simulink model "PlantWateringProject"  (R2024a)
settings: Solver=VariableStepAuto  StartTime=0.0  StopTime=120.0  RelTol=1e-3
settings Model: Creator=charlieperkins  LastModifiedBy=charlieperkins

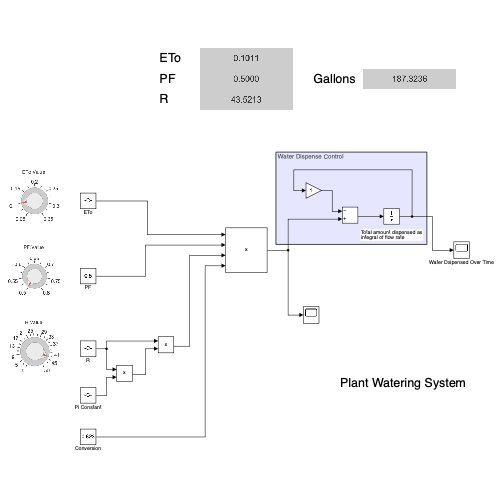
[thumbnail: Simulink's stored preview of the top-level diagram]
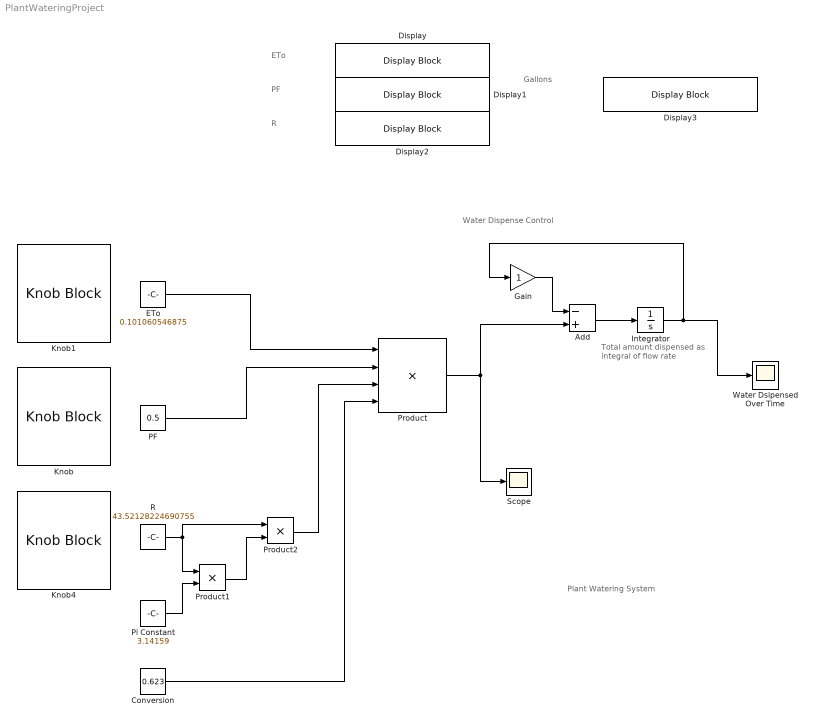
== system PlantWateringProject ==
  note: Water Dispense Control
  note: Total amount dispensed as
      | integral of flow rate
  note: ETo
  note: PF
  note: R
  note: Gallons
  note: Plant Watering System
  Add : Sum  Inputs=-+
  Conversion : Constant  Value=0.623
  Display{,1..3} (4 alike) : DisplayBlock  LabelPosition=Hide  Transparency=1
  ETo : Constant  Value=0.101060546875
  Gain : Gain
  Integrator : Integrator
  Knob : KnobBlock  ScaleMin=0.5  ScaleMax=0.8
  Knob1 : KnobBlock  ScaleMin=0.05  ScaleMax=0.35
  Knob4 : KnobBlock  ScaleMin=1  ScaleMax=50
  PF : Constant  Value=0.5
  Pi Constant : Constant  Value=3.14159
  Product : Product  Inputs=4
  Product1 : Product
  Product2 : Product
  R : Constant  Value=43.52128224690755
  Scope : Scope
  Water Dsipensed Over Time : Scope
  wires:
  Product/1 -> Add/2, Scope/1
  Integrator/1 -> Water Dsipensed Over Time/1, Gain/1
  Gain/1 -> Add/1
  Add/1 -> Integrator/1
  Conversion/1 -> Product/4
  ETo/1 -> Product/1
  PF/1 -> Product/2
  Pi Constant/1 -> Product1/2
  R/1 -> Product1/1, Product2/1
  Product1/1 -> Product2/2
  Product2/1 -> Product/3
